simulink model "Template_Controller"  (R2019b)
settings: Solver=VariableStepAuto  StartTime=0.0  StopTime=10.0  RelTol=1e-3
settings Model: Creator=Duin home  LastModifiedBy=Duin home

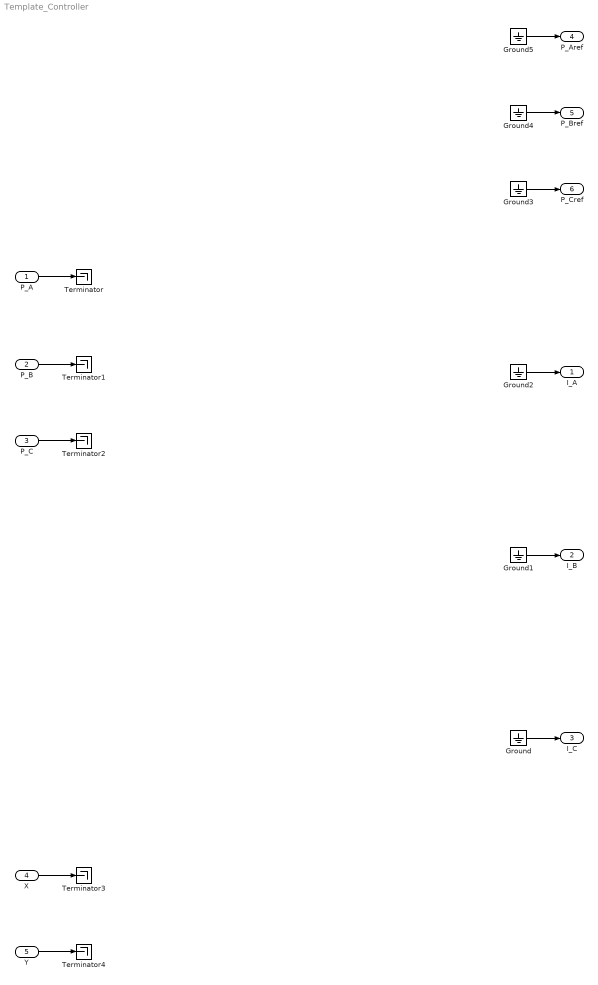
== system Template_Controller ==
  P_A : Inport
  P_B : Inport  Port=2
  P_C : Inport  Port=3
  X : Inport  Port=4
  Y : Inport  Port=5
  Ground{,1..5} (6 alike) : Ground
  Terminator{,1..4} (5 alike) : Terminator
  I_A : Outport
  I_B : Outport  Port=2
  I_C : Outport  Port=3
  P_Aref : Outport  Port=4
  P_Bref : Outport  Port=5
  P_Cref : Outport  Port=6
  wires:
  P_A/1 -> Terminator/1
  P_B/1 -> Terminator1/1
  P_C/1 -> Terminator2/1
  X/1 -> Terminator3/1
  Y/1 -> Terminator4/1
  Ground/1 -> I_C/1
  Ground1/1 -> I_B/1
  Ground2/1 -> I_A/1
  Ground3/1 -> P_Cref/1
  Ground4/1 -> P_Bref/1
  Ground5/1 -> P_Aref/1
